simulink model "RTS_szabalyzo"  (R2018a)
settings: Solver=FixedStepDiscrete  StartTime=0.0  StopTime=100  FixedStep=0.5  RelTol=1e-3  EnableMultiTasking=on
values from neighbouring files (symbols this model uses):
  a0 = 0.6065    [Parameters.m]    (also in RTS_sf.m = u(6))
  a1 = -1.4138    [Parameters.m]    (also in RTS_sf.m = u(5))
  am0 = 0.4966    [Parameters.m]    (also in RTS_sf.m)
  am1 = -1.3205    [Parameters.m]    (also in RTS_sf.m)
  b0 = 0.0883    [Parameters.m]    (also in RTS_sf.m = u(8))
  b1 = 0.1044    [Parameters.m]    (also in RTS_sf.m = u(7))
  bm1 = 0.1761    [Parameters.m]    (also in RTS_sf.m)
settings Model: Creator=kiss-miki.t  LastModifiedBy=Turing
settings DataIOCC: LimitDataPoints=on  SaveFormat=Array
settings OptimizationCC: LifeSpan=inf
settings DebuggingCC: SolverPrmCheckMsg=warning  SFUnexpectedBacktrackingDiag=warning  SFNoUnconditionalDefaultTransitionDiag=warning  SFExecutionAtInitializationDiag=none
settings HardwareCC: ProdBitPerPointer=32  ProdBitPerSizeT=32  ProdBitPerPtrDiffT=32  ProdLargestAtomicFloat=None  ProdIntDivRoundTo=Undefined  ProdEndianess=Unspecified  ProdWordSize=32  ProdHWDeviceType=32-bit Generic
settings ModelReferenceCC: PropagateSignalLabelsOutOfModel=off
settings CodeAppCC: StateflowObjectComments=on
settings GRTTargetCC: TargetLangStandard=C89/C90 (ANSI)  GeneratePreprocessorConditionals=Disable all
settings ConfigComp: CovMetricSettings=dw  CovHtmlReporting=on  CovSaveCumulativeToWorkspaceVar=on  CovSaveSingleToWorkspaceVar=on  CovExternalEMLEnable=off  CovSFcnEnable=off

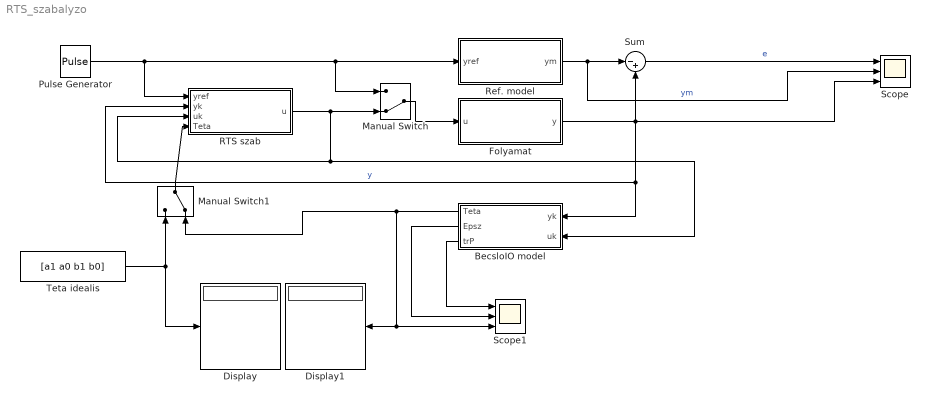
== system RTS_szabalyzo ==
  BecsloIO model : Subsystem
  Display : Display
  Display1 : Display
  Folyamat : Subsystem
  Manual Switch : ManualSwitch  CurrentSetting=0
  Manual Switch1 : ManualSwitch  CurrentSetting=0
  Pulse Generator : DiscretePulseGenerator  Amplitude=10  Period=100  PulseWidth=50  SampleTime=0.5
  RTS szab : Subsystem
  Ref. model : Subsystem
  Scope : Scope  NumInputPorts=3
  Scope1 : Scope  NumInputPorts=3
  Sum : Sum  Inputs=|-+
  Teta idealis : Constant  Value=[a1 a0 b1 b0]
  wires:
  Folyamat/1(y) -> Scope/3, Sum/2, BecsloIO model/1(yk), RTS szab/2(yk)  "y"
  Sum/1 -> Scope/1  "e"
  Pulse Generator/1 -> RTS szab/1(yref), Manual Switch/1, Ref. model/1(yref)
  RTS szab/1(u) -> BecsloIO model/2(uk), RTS szab/3(uk), Manual Switch/2
  Manual Switch/1 -> Folyamat/1(u)
  Teta idealis/1 -> Display/1, Manual Switch1/1
  BecsloIO model/1(Teta) -> Scope1/3, Display1/1, Manual Switch1/2
  Manual Switch1/1 -> RTS szab/4(Teta)
  BecsloIO model/2(Epsz) -> Scope1/2
  BecsloIO model/3("trP ") -> Scope1/1
  Ref. model/1(ym) -> Scope/2, Sum/1  "ym"

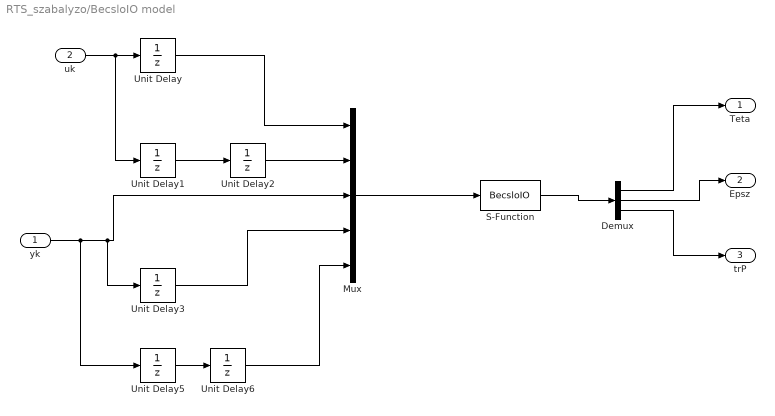
== system RTS_szabalyzo/BecsloIO model ==
  yk : Inport
  uk : Inport  Port=2
  Demux : Demux  Outputs=[4 1 1]
  Mux : Mux  Inputs=5
  S-Function : S-Function  FunctionName=BecsloIO  SFunctionDeploymentMode=off  EnableBusSupport=off
  Unit Delay{,1..3,5..6} (6 alike) : UnitDelay  SampleTime=0.5
  Teta : Outport
  Epsz : Outport  Port=2
  "trP " : Outport  Port=3
  wires:
  uk/1 -> Unit Delay1/1, Unit Delay/1
  Unit Delay/1 -> Mux/1
  Unit Delay2/1 -> Mux/2
  Unit Delay1/1 -> Unit Delay2/1
  yk/1 -> Unit Delay5/1, Unit Delay3/1, Mux/3
  Unit Delay3/1 -> Mux/4
  Unit Delay5/1 -> Unit Delay6/1
  Unit Delay6/1 -> Mux/5
  Mux/1 -> S-Function/1
  S-Function/1 -> Demux/1
  Demux/1 -> Teta/1
  Demux/2 -> Epsz/1
  Demux/3 -> "trP "/1

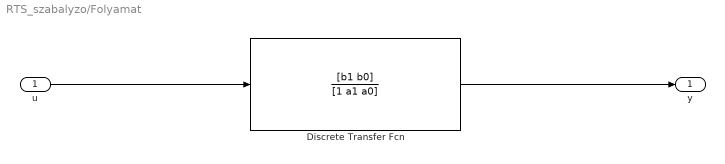
== system RTS_szabalyzo/Folyamat ==
  u : Inport
  Discrete Transfer Fcn : DiscreteTransferFcn  Numerator=[b1 b0]  Denominator=[1 a1 a0]  SampleTime=0.5
  y : Outport
  wires:
  u/1 -> Discrete Transfer Fcn/1
  Discrete Transfer Fcn/1 -> y/1

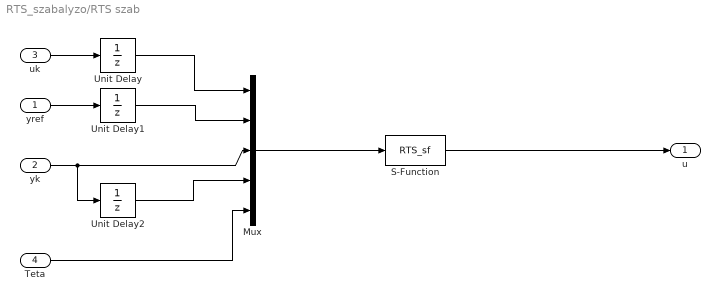
== system RTS_szabalyzo/RTS szab ==
  yref : Inport
  yk : Inport  Port=2
  uk : Inport  Port=3
  Teta : Inport  Port=4
  Mux : Mux  Inputs=5
  S-Function : S-Function  FunctionName=RTS_sf  SFunctionDeploymentMode=off  EnableBusSupport=off
  Unit Delay : UnitDelay  SampleTime=0.5
  Unit Delay1 : UnitDelay  SampleTime=0.5
  Unit Delay2 : UnitDelay  SampleTime=0.5
  u : Outport
  wires:
  Mux/1 -> S-Function/1
  S-Function/1 -> u/1
  uk/1 -> Unit Delay/1
  Unit Delay/1 -> Mux/1
  yref/1 -> Unit Delay1/1
  Unit Delay1/1 -> Mux/2
  yk/1 -> Unit Delay2/1, Mux/3
  Teta/1 -> Mux/5
  Unit Delay2/1 -> Mux/4

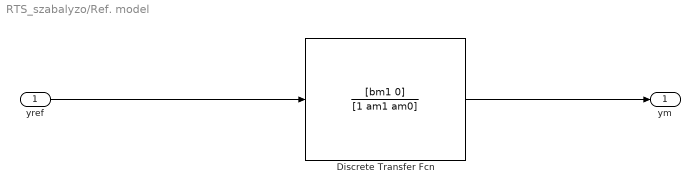
== system RTS_szabalyzo/Ref. model ==
  yref : Inport
  Discrete Transfer Fcn : DiscreteTransferFcn  Numerator=[bm1 0]  Denominator=[1 am1 am0]  SampleTime=0.5
  ym : Outport
  wires:
  yref/1 -> Discrete Transfer Fcn/1
  Discrete Transfer Fcn/1 -> ym/1
